simulink model "simulink_model_example"  (R2024b)
settings: Solver=FixedStepDiscrete  StartTime=0.0  StopTime=10.0  RelTol=1e-3
settings DataIOCC: SignalLogging=off  SaveTime=off

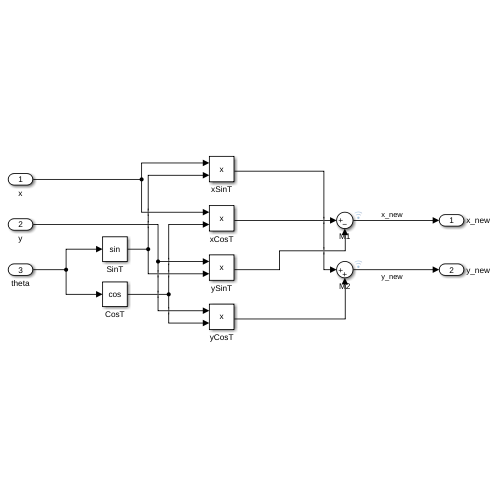
[thumbnail: Simulink's stored preview of the top-level diagram]
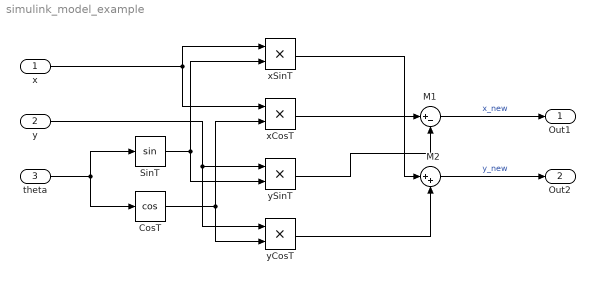
== system simulink_model_example ==
  x : Inport
  y : Inport  Port=2
  theta : Inport  Port=3
  CosT : Trigonometry  Operator=cos
  M1 : Sum  Inputs=|+-
  M2 : Sum  Inputs=|++
  SinT : Trigonometry
  xCosT : Product
  xSinT : Product
  yCosT : Product
  ySinT : Product
  Out1 : Outport  SignalName=x_new
  Out2 : Outport  Port=2  SignalName=y_new
  wires:
  theta/1 -> CosT/1, SinT/1
  CosT/1 -> yCosT/2, xCosT/2
  x/1 -> xSinT/1, xCosT/1
  SinT/1 -> ySinT/2, xSinT/2
  y/1 -> yCosT/1, ySinT/1
  xCosT/1 -> M1/1
  ySinT/1 -> M1/2
  xSinT/1 -> M2/1
  yCosT/1 -> M2/2
  M1/1 -> Out1/1  "x_new"
  M2/1 -> Out2/1  "y_new"
